simulink model "cartPoleModel"  (R2023b)
settings: Solver=VariableStepAuto  StartTime=0.0  StopTime=10.0  RelTol=1e-3
undefined symbols (not defined in the file): A, B, x0
settings Model: Creator=rodrigoscott  LastModifiedBy=rodrigoscott

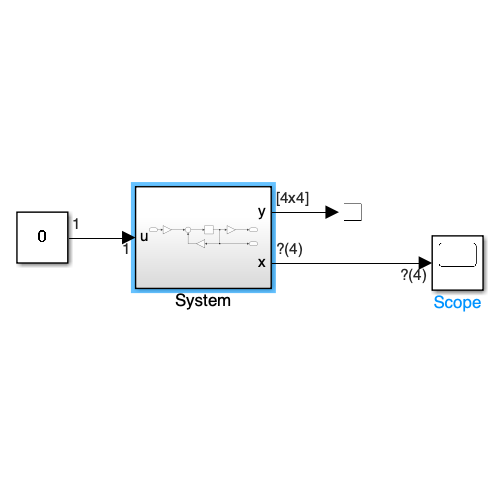
[thumbnail: Simulink's stored preview of the top-level diagram]
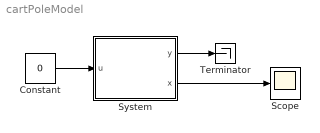
== system cartPoleModel ==
  Constant : Constant  Value=0
  Scope : Scope
  System : Subsystem
  Terminator : Terminator
  wires:
  Constant/1 -> System/1(u)
  System/1(y) -> Terminator/1
  System/2(x) -> Scope/1

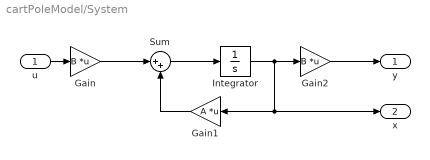
== system cartPoleModel/System ==
  u : Inport
  Gain : Gain  Gain=B  Multiplication=Matrix(K*u)
  Gain1 : Gain  Gain=A  Multiplication=Matrix(K*u)
  Gain2 : Gain  Gain=B  Multiplication=Matrix(K*u)
  Integrator : Integrator  InitialCondition=x0
  Sum : Sum  Inputs=|++
  y : Outport
  x : Outport  Port=2
  wires:
  Gain2/1 -> y/1
  Sum/1 -> Integrator/1
  Integrator/1 -> Gain2/1, x/1, Gain1/1
  Gain/1 -> Sum/1
  u/1 -> Gain/1
  Gain1/1 -> Sum/2
